simulink model "LR6"  (R2023b)
settings: Solver=VariableStepAuto  StartTime=0.0  StopTime=100  MaxStep=0.01  RelTol=1e-3
values from neighbouring files (symbols this model uses):
  a0 = ae0*ap0    (= 0.01)    [mL6.m]
  a1 = ae0*ap1 + ap0    (= 0.06)    [mL6.m]
  a2 = ae0+ap1    (= 0.33)    [mL6.m]
  Ac = [  0   1   0 ... (first row only)    [mL6.m]
  Acm = [ Ae,         0, 0 ... (first row only)    [mL6.m]
  Ae = [ -ae0]    [mL6.m]
  ae0 = 1/T1    (= 0.25)    [mL6.m]
  Ap = [ 0 1 ;  -ap0  -ap1 ]    [mL6.m]
  ap0 = 1 / (T2*T2)    (= 0.04)    [mL6.m]
  ap1 = 2*q / T2    (= 0.08)    [mL6.m]
  b0 = be0*K2*bp0    (= 0.0005)    [mL6.m]
  b1 = be0*K2*bp1    (= 0.0005)    [mL6.m]
  Bc = [  0 ... (first row only)    [mL6.m]
  Bcm = [[0; Bpf],  [Be; 0; 0] ]    [mL6.m]
  Be = [ 1 ]    [mL6.m]
  be0 = K1/T1    (= 0.125)    [mL6.m]
  bp0 = 1 / (T2*T2)    (= 0.04)    [mL6.m]
  bp1 = T3 / (T2*T2)    (= 0.04)    [mL6.m]
  Bpf = [ 0 ; 1 ]    [mL6.m]
  Bpr = [ 0 ; K2 ]    [mL6.m]
  Cc = [ b0   b1   0 ]    [mL6.m]
  Ccm = [[0 Cp]; [Ce 0 0]]    [mL6.m]
  Cd = [ n0   n1   n2 ]    [mL6.m]
  Ce = [ be0]    [mL6.m]
  Cp = [ bp0   bp1  ]    [mL6.m]
  Dc = 0    [mL6.m]
  De = 0    [mL6.m]
  Dp = [0 0]    [mL6.m]
  K1 = 0.5    [mL6.m]
  K2 = 0.1    [mL6.m]
  m0 = Wzoh_plant.Denominator{1}(4)    [mL6.m]
  m1 = Wzoh_plant.Denominator{1}(3)    [mL6.m]
  m2 = Wzoh_plant.Denominator{1}(2)    [mL6.m]
  n0 = Wzoh_plant.Numerator{1}(4)    [mL6.m]
  n1 = Wzoh_plant.Numerator{1}(3)    [mL6.m]
  n2 = Wzoh_plant.Numerator{1}(2)    [mL6.m]
  q = 0.2    [mL6.m]
  T1 = 4    [mL6.m]
  T2 = 5    [mL6.m]
  T3 = 1    [mL6.m]
  Ts = 0.1* (T1 + T2 + T3)    (= 1)    [mL6.m]
  Un = 80    [mL6.m]
settings Model: Creator=td  LastModifiedBy=killer
settings SolverCC: AlgebraicLoopSolver=TrustRegion
settings DataIOCC: ReturnWorkspaceOutputs=off
settings DebuggingCC: UnconnectedInputMsg=warning  UnconnectedOutputMsg=warning  UnconnectedLineMsg=warning  ArithmeticOperatorsInVariantConditions=warning
settings ModelReferenceCC: EnableRefExpFcnMdlSchedulingChecks=on
settings SFSimCC: CustomCodeUndefinedFunction=UseInterfaceOnly

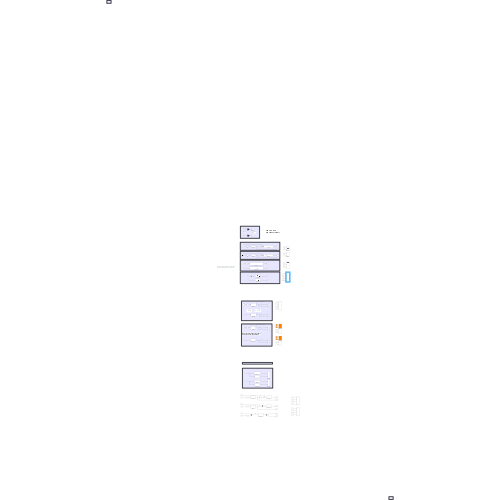
[thumbnail: Simulink's stored preview of the top-level diagram]
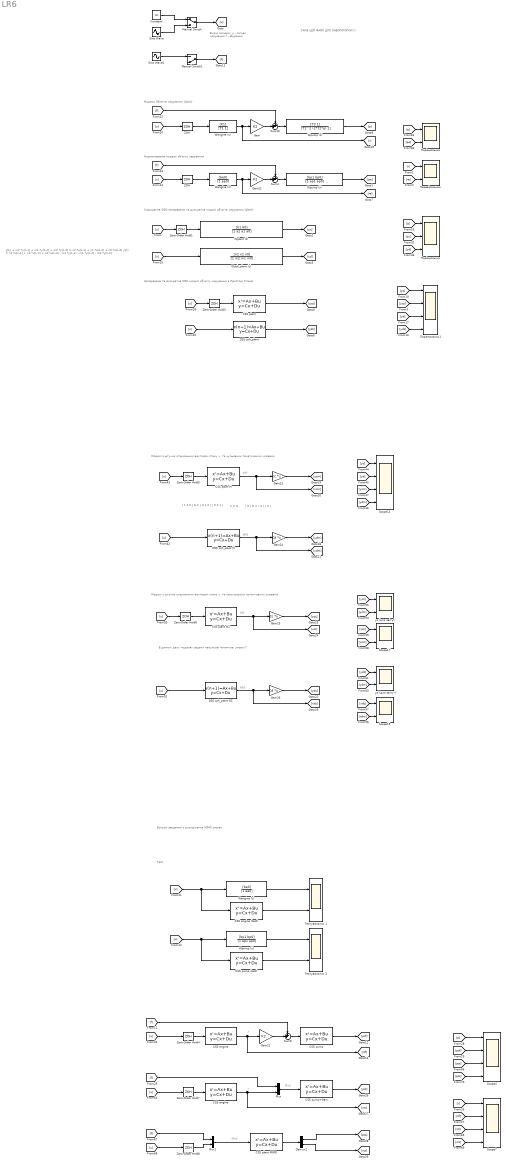
== system LR6 ==
  note: Бонусні завдання з дослідження MIMO систем
  note: r
  note: [f;r]
  note: Test
  note: В данних двох моделях задати
      | ненульові початкові умови!!!
  note: Моделі з штучно отриманним вектором стану х, та ненульовими початковими умовами
  note: Моделі з штучно отриманним вектором стану х, та нульовими початковими умовами
  note: Спрощенна SISO неперервна та дискретна моделі об’єкта керування (plant)
  note: Модель Об'єкта керування (plant)
  note: Вхідні сигнали:
      |
      | u - сигнал керування
      |
      | f - збурення
  note: x(t)
  note: y[k] + m2 *y[k-1] + m1 *y[k-2] + m0 *y[k-3] = n2 *u[k-1] + n1 *u[k-2] + n0 *u[k-3]
      |
      | y[k] = n2 *u[k-1] + n1 *u[k-2] + n0 *u[k-3] - m2 *y[k-1] - m1 *y[k-2] - m0 *y[k-3]
  note: [ 1 0 0 ]
      | E = [ 0 1 0 ]
      | [ 0 0 1 ]
  note: x[k]
  note: C = E,
  note: [ 0 ]
      | D = [ 0 ]
      | [ 0 ]
  note: x[k]
  note: x(t)
  note: Нормалізована модель об'єкту керування
  note: Неперервна та дискретна SISO моделі об’єкту керування в Просторі Станів
  note: r
  note: [f;u]
  note: САМЕ ЦЕЙ ФАЙЛ
      | ДЛЯ ЛАБОРАТОРКИ!!!!
  "  Wpump (s)" : TransferFcn  Numerator=[T3 1]  Denominator=[T2^2 (2*T2*q) 1]
  " ZOH " : ZeroOrderHold  SampleTime=Ts
  " Перевіряльник " : Scope  NumInputPorts=2
  " Порівняльник " : Scope  NumInputPorts=2
  CSS engine : StateSpace  A=Ae  B=Be  C=Ce  D=De  InitialCondition=0
  "CSS engine " : StateSpace  A=Ae  B=Be  C=Ce  D=De  InitialCondition=0
  CSS engine (test) : StateSpace  A=Ae  B=Be  C=Ce  D=0  InitialCondition=0
  CSS plant : StateSpace  A=Ac  B=Bc  C=Cc  D=Dc  InitialCondition=[8000;0;0]
  CSS plant M : StateSpace  A="[ 0 1 0 ; 0 0 1 ;  -a0  -a1  -a2 ]"  B=[ 0 ; 0 ; 1 ]  C=eye(3)  D=[0; 0; 0]  InitialCondition=0
  CSS plant MIMO : StateSpace  A=Acm  B=Bcm  C=Ccm  D=[0 0; 0 0]  InitialCondition=0
  CSS plant NZ : StateSpace  A="[ 0 1 0 ; 0 0 1 ;  -a0  -a1  -a2 ]"  B=[ 0 ; 0 ; 1 ]  C=eye(3)  D=[0; 0; 0]  InitialCondition=[5915; 0; 0 ]
  CSS pump : StateSpace  A=Ap  B=[ 0 ; 1 ]  C=Cp  D=0  InitialCondition=0
  CSS pump (test) : StateSpace  A=Ap  B=[ 0 ; 1 ]  C=Cp  D=0  InitialCondition=0
  CSS pump+Gain : StateSpace  A=Ap  B="[Bpf  Bpr]"  C=Cp  D=Dp  InitialCondition=0
  Constant : Constant  Value=Un
  DSS zoh_plant : DiscreteStateSpace  A="[ 0 1 0 ; 0 0 1 ;  -m0  -m1  -m2 ]"  B=[ 0 ; 0 ; 1 ]  C="[ n0   n1   n2 ]"  D=0  InitialCondition=[9439.5;; 9439.5; 9439.5]  SampleTime=Ts
  DSS zoh_plant M : DiscreteStateSpace  A="[ 0 1 0 ; 0 0 1 ;  -m0  -m1  -m2 ]"  B=[ 0 ; 0 ; 1 ]  C=[1 0 0; 0 1 0; 0 0 1]  D=[0;0;0]  SampleTime=Ts
  DSS zoh_plant NZ : DiscreteStateSpace  A="[ 0 1 0 ; 0 0 1 ;  -m0  -m1  -m2 ]"  B=[ 0 ; 0 ; 1 ]  C=[1 0 0; 0 1 0; 0 0 1]  D=[0;0;0]  InitialCondition="[5412.7; 5412.7; 5412.7  ]"  SampleTime=Ts
  Demux2 : Demux  Outputs=2
  Gain : Gain  Gain=K2
  Gain21 : Gain  Gain=K2
  Gain22 : Gain  Gain=K2
  Gain23 : Gain  Gain=Cc  Multiplication=Matrix(K*u)
  Gain24 : Gain  Gain=Cd  Multiplication=Matrix(K*u)
  Gain25 : Gain  Gain=Cc  Multiplication=Matrix(K*u)
  Gain26 : Gain  Gain=Cd  Multiplication=Matrix(K*u)
  Manual Switch : ManualSwitch
  Manual Switch1 : ManualSwitch  CurrentSetting=0
  Mux : Mux  Inputs=2
  Mux1 : Mux  Inputs=2
  Scope13 : Scope  NumInputPorts=4
  Scope17 : Scope  NumInputPorts=2
  Scope19 : Scope  NumInputPorts=2
  Scope4 : Scope  NumInputPorts=4
  Scope7 : Scope  NumInputPorts=4
  Sine Wave : Sin  Frequency=0.4  SampleTime=0
  Sine Wave1 : Sin  Amplitude=5  Frequency=0.4  SampleTime=Ts
  Sum10 : Sum  Inputs=++|
  Sum4 : Sum  Inputs=++|
  Sum5 : Sum  Inputs=++|
  Wengine (s) : TransferFcn  Numerator=[be0]  Denominator=[1 ae0]
  "Wengine (s) " : TransferFcn  Numerator=[K1]  Denominator=[T1 1]
  "Wengine (s)   " : TransferFcn  Numerator=[be0]  Denominator=[1 ae0]
  Wplant (s) : TransferFcn  Numerator=[b1 b0]  Denominator=[1 a2 a1 a0]
  Wpump (s) : TransferFcn  Numerator=[bp1 bp0]  Denominator=[1 ap1 ap0]
  "Wpump (s)  " : TransferFcn  Numerator=[bp1 bp0]  Denominator=[1 ap1 ap0]
  Wzoh_plant (z) : DiscreteTransferFcn  Numerator=[n2 n1 n0]  Denominator=[1 m2 m1 m0]  SampleTime=Ts
  ZOH : ZeroOrderHold  SampleTime=Ts
  Zero-Order Hold{1,3..8} (7 alike) : ZeroOrderHold  SampleTime=Ts
  "yc (для звіту!) " : Scope  NumInputPorts=2
  "yd (для звіту!) " : Scope  NumInputPorts=2
  Порівняльник : Scope  NumInputPorts=3
  Порівняльник1 : Scope  NumInputPorts=4
  Тестувальник 1 : Scope  NumInputPorts=2
  Тестувальник 2 : Scope  NumInputPorts=2
  wires:
  Manual Switch/1 -> [u]
  Constant/1 -> Manual Switch/1
  Sine Wave/1 -> Manual Switch/2
  [u] -> Zero-Order Hold1/1
  Wpump (s)/1 -> [pe]
  Wplant (s)/1 -> [yc]
  Wzoh_plant (z)/1 -> [yd]
  DSS zoh_plant/1 -> [yds]
  [u] -> DSS zoh_plant/1
  Zero-Order Hold1/1 -> Wplant (s)/1
  Wengine (s)/1 -> Gain21/1, [re]
  " ZOH "/1 -> Wengine (s)/1
  [u] -> " ZOH "/1
  [u] -> Wzoh_plant (z)/1
  CSS plant/1 -> [ycs]
  "  Wpump (s)"/1 -> [p]
  ZOH/1 -> "Wengine (s) "/1
  [u] -> ZOH/1
  [u] -> Zero-Order Hold3/1
  Zero-Order Hold3/1 -> CSS plant/1
  "Wengine (s) "/1 -> Gain/1, [r]
  [f] -> Sum10/1
  Manual Switch1/1 -> [f]
  Sine Wave1/1 -> Manual Switch1/1
  Sum4/1 -> Wpump (s)/1
  [f] -> Sum4/1
  Zero-Order Hold4/1 -> CSS engine/1
  CSS engine/1 -> Gain22/1, [rcf]
  [f] -> Sum5/1
  Sum5/1 -> CSS pump/1
  "Wpump (s)  "/1 -> Тестувальник 2/1
  [u] -> CSS pump (test)/1, "Wpump (s)  "/1
  CSS pump (test)/1 -> Тестувальник 2/2
  [u] -> Zero-Order Hold4/1
  CSS pump/1 -> [pcf]
  [r] -> Scope7/1
  [rcf] -> Scope7/2
  [pcf] -> Scope4/2
  [p] -> Scope4/1
  Gain21/1 -> Sum4/2
  Sum10/1 -> "  Wpump (s)"/1
  Gain/1 -> Sum10/2
  Gain22/1 -> Sum5/2
  [u] -> DSS zoh_plant M/1
  [u] -> Zero-Order Hold5/1
  Zero-Order Hold5/1 -> CSS plant M/1
  CSS plant M/1 -> [xcm], Gain23/1
  Gain23/1 -> [ycm]
  DSS zoh_plant M/1 -> [xdm], Gain24/1
  Gain24/1 -> [ydm]
  [ycm] -> Scope13/3
  [yc] -> Scope13/1
  [yd] -> Scope13/2
  [ydm] -> Scope13/4
  Zero-Order Hold6/1 -> CSS plant NZ/1
  [u] -> DSS zoh_plant NZ/1
  [u] -> Zero-Order Hold6/1
  Gain26/1 -> [ydz]
  DSS zoh_plant NZ/1 -> [xdz], Gain26/1
  CSS plant NZ/1 -> [xcz], Gain25/1
  Gain25/1 -> [ycz]
  [ydz] -> "yd (для звіту!) "/1
  [ydm] -> "yd (для звіту!) "/2
  [xcm] -> Scope17/2
  [xcz] -> Scope17/1
  [ycz] -> "yc (для звіту!) "/1
  [ycm] -> "yc (для звіту!) "/2
  [xdz] -> Scope19/1
  [xdm] -> Scope19/2
  [p] -> " Порівняльник "/1
  [pe] -> " Порівняльник "/2
  [r] -> " Перевіряльник "/1
  [re] -> " Перевіряльник "/2
  [yd] -> Порівняльник/3
  [yc] -> Порівняльник/2
  [p] -> Порівняльник/1
  [ycs] -> Порівняльник1/2
  [yds] -> Порівняльник1/4
  [yd] -> Порівняльник1/3
  [yc] -> Порівняльник1/1
  CSS engine (test)/1 -> Тестувальник 1/2
  "Wengine (s)   "/1 -> Тестувальник 1/1
  [u] -> CSS engine (test)/1, "Wengine (s)   "/1
  Zero-Order Hold7/1 -> "CSS engine "/1
  [f] -> Mux/1
  [u] -> Zero-Order Hold7/1
  CSS pump+Gain/1 -> [pct]
  "CSS engine "/1 -> Mux/2, [rct]
  [rct] -> Scope7/3
  [pct] -> Scope4/3
  Mux/1 -> CSS pump+Gain/1
  [rcs] -> Scope7/4
  [pcs] -> Scope4/4
  [u] -> Zero-Order Hold8/1
  Mux1/1 -> CSS plant MIMO/1
  [f] -> Mux1/1
  Demux2/1 -> [pcs]
  Zero-Order Hold8/1 -> Mux1/2
  CSS plant MIMO/1 -> Demux2/1
  Demux2/2 -> [rcs]
